simulink model "semi_solarwind"  (R2023b)
settings: Solver=VariableStepAuto  StartTime=0.0  StopTime=5  RelTol=1e-3
undefined symbols (not defined in the file): D1, Delta, Ion, Lithium
libraries: spsSeriesRLCBranchLib x26, spsVoltageMeasurementLib x9, spsDiodeLib x8, dspsrcs4 x8, spsCurrentMeasurementLib x5, spsThreePhaseVIMeasurementLib x5, spsMosfetLib x4, spsPWMGeneratorDCDCLib x4, spsPVArrayLib x4, spsThreePhaseTransformerTwoWindingsLib x3, spsThreePhaseParallelRLCLoadLib x3, spsThreePhaseSeriesRLCBranchLib x3
(part 1 of 2)
settings Model: Creator=yeowy  LastModifiedBy=yeowy

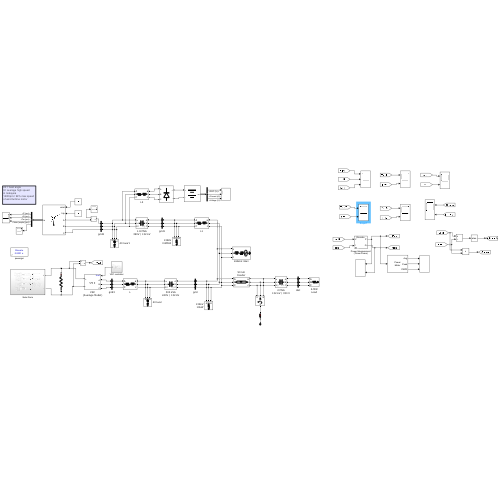
[thumbnail: Simulink's stored preview of the top-level diagram]
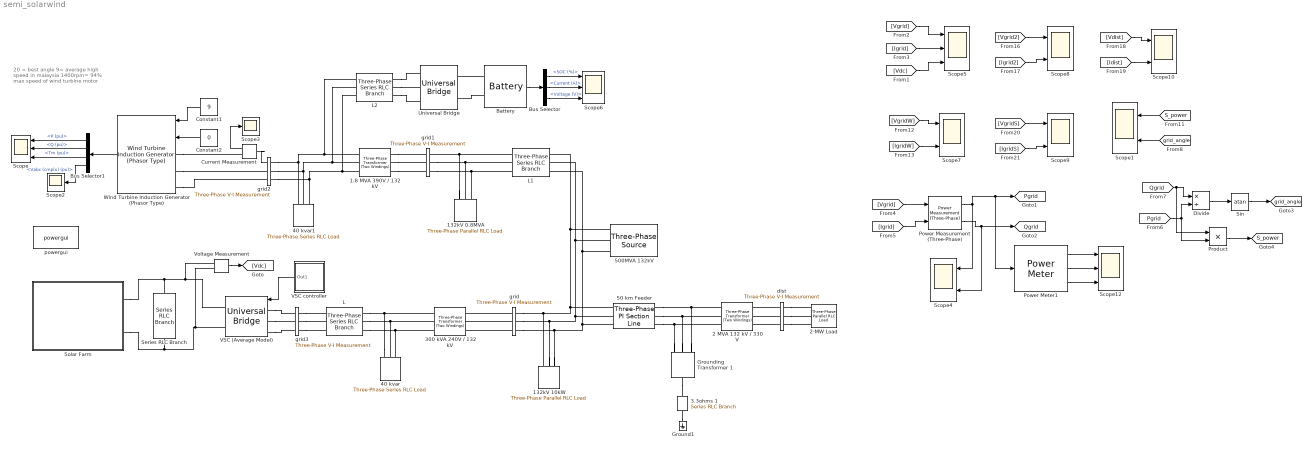
== system semi_solarwind ==
  note: 20 = best angle
      | 9= average high speed
      | in malaysia
      | 1400rpm= 94% max speed
      | of wind turbine motor
  1.8 MVA 390V / 132 kV : spsThreePhaseTransformerTwoWindingsLib/Three-Phase Transformer (Two Windings)  Winding1Connection=Yg  Winding2Connection=Delta (D1)  CoreType=Three single-phase transformers  SetSaturation=off  Hysteresis=off  DataFile='hysteresis'  SetInitialFlux=off  Measurements=None  UNITS=pu  NominalPower=[1.8e6 , 50 ]  Winding1=[ 132e3 , 0.001 , 0.03 ]  Winding2=[ 390 , 0.001 , 0.03 ]  Rm=500  Lm=500  L0=0.5  Saturation=[ 0,0 ; 0.0024,1.2 ; 1.0,1.52 ]  InitialFluxes=[ 0.8 , -0.8 , 0.7 ]  BreakLoop=off  DiscreteSolver=Trapezoidal iterative  DataType=off  TransfoNumber=0
  132kV 0.8MVA : spsThreePhaseParallelRLCLoadLib/Three-Phase Parallel RLC Load  LConnTagsString=A|B|C  Configuration=Y (grounded)  NominalVoltage=132e3  Vabc=[1e3 1e3 1e3]  Vabcp=[1e3 1e3 1e3]  NominalFrequency=50  UnbalancedPower=off  ActivePower=0.8e6  InductivePower=0  CapacitivePower=0  Pabc=[10e3 9e3 11e3]  QLabc=[100 90 110]  QCabc=[100 90 110]  Pabcp=[10e3 9e3 11e3]  QLabcp=[100 90 110]  QCabcp=[100 90 110]  Measurements=None  LoadType=constant Z
  132kV 10kW : spsThreePhaseParallelRLCLoadLib/Three-Phase Parallel RLC Load  LConnTagsString=A|B|C  Configuration=Y (grounded)  NominalVoltage=132e3  Vabc=[1e3 1e3 1e3]  Vabcp=[1e3 1e3 1e3]  NominalFrequency=50  UnbalancedPower=off  ActivePower=10e3  InductivePower=0  CapacitivePower=0  Pabc=[10e3 9e3 11e3]  QLabc=[100 90 110]  QCabc=[100 90 110]  Pabcp=[10e3 9e3 11e3]  QLabcp=[100 90 110]  QCabcp=[100 90 110]  Measurements=None  LoadType=constant Z
  2 MVA 132 kV / 330 V : spsThreePhaseTransformerTwoWindingsLib/Three-Phase Transformer (Two Windings)  Winding1Connection=Delta (D1)  Winding2Connection=Yg  CoreType=Three single-phase transformers  SetSaturation=off  Hysteresis=off  DataFile='hysteresis'  SetInitialFlux=off  Measurements=None  UNITS=pu  NominalPower=[2e6 , 50 ]  Winding1=[ 330 , 0.001 , 0.03 ]  Winding2=[ 132e3 , 0.001 , 0.03 ]  Rm=500  Lm=500  L0=0.5  Saturation=[ 0,0 ; 0.0024,1.2 ; 1.0,1.52 ]  InitialFluxes=[0.79999 -0.79999 0.70002]  BreakLoop=off  DiscreteSolver=Trapezoidal iterative  DataType=off  TransfoNumber=0
  2-MW Load : spsThreePhaseParallelRLCLoadLib/Three-Phase Parallel RLC Load  LConnTagsString=A|B|C  Configuration=Y (grounded)  NominalVoltage=240  Vabc=[1e3 1e3 1e3]  Vabcp=[1e3 1e3 1e3]  NominalFrequency=50  UnbalancedPower=off  ActivePower=2e6  InductivePower=0  CapacitivePower=0  Pabc=[10e3 9e3 11e3]  QLabc=[100 90 110]  QCabc=[100 90 110]  Pabcp=[10e3 9e3 11e3]  QLabcp=[100 90 110]  QCabcp=[100 90 110]  Measurements=None  LoadType=constant Z
  3.3ohms 1 : spsSeriesRLCBranchLib/Series RLC Branch  LConnTagsString=__new0  RConnTagsString=__new0  BranchType=R  Resistance=3.3  Inductance=[]  SetiL0=off  InitialCurrent=0  Capacitance=[]  Setx0=off  InitialVoltage=0  Measurements=None
  300 kVA 240V / 132 kV : spsThreePhaseTransformerTwoWindingsLib/Three-Phase Transformer (Two Windings)  Winding1Connection=Yg  Winding2Connection=Delta (D1)  CoreType=Three single-phase transformers  SetSaturation=off  Hysteresis=off  DataFile='hysteresis'  SetInitialFlux=off  Measurements=None  UNITS=pu  NominalPower=[0.3e6 , 50 ]  Winding1=[ 132e3 , 0.001 , 0.03 ]  Winding2=[ 240 , 0.001 , 0.03 ]  Rm=500  Lm=500  L0=0.5  Saturation=[ 0,0 ; 0.0024,1.2 ; 1.0,1.52 ]  InitialFluxes=[ 0.8 , -0.8 , 0.7 ]  BreakLoop=off  DiscreteSolver=Trapezoidal iterative  DataType=off  TransfoNumber=0
  40 kvar : spsThreePhaseSeriesRLCLoadLib/Three-Phase Series RLC Load  LConnTagsString=A|B|C  Configuration=Y (grounded)  NominalVoltage=240  Vabc=[1e3 1e3 1e3]  Vabcp=[1e3 1e3 1e3]  NominalFrequency=50  UnbalancedPower=off  ActivePower=400  InductivePower=0  CapacitivePower=400  Pabc=[10e3 9e3 11e3]  QLabc=[100 90 110]  QCabc=[100 90 110]  Pabcp=[10e3 9e3 11e3]  QLabcp=[100 90 110]  QCabcp=[100 90 110]  Measurements=None  LoadType=constant Z
  40 kvar1 : spsThreePhaseSeriesRLCLoadLib/Three-Phase Series RLC Load  LConnTagsString=A|B|C  Configuration=Y (grounded)  NominalVoltage=240  Vabc=[1e3 1e3 1e3]  Vabcp=[1e3 1e3 1e3]  NominalFrequency=50  UnbalancedPower=off  ActivePower=400  InductivePower=0  CapacitivePower=40e3  Pabc=[10e3 9e3 11e3]  QLabc=[100 90 110]  QCabc=[100 90 110]  Pabcp=[10e3 9e3 11e3]  QLabcp=[100 90 110]  QCabcp=[100 90 110]  Measurements=None  LoadType=constant Z
  50 km Feeder : spsThreePhasePISectionLineLib/Three-Phase PI Section Line  LConnTagsString=a|b|c  RConnTagsString=A|B|C  Length=50  Frequency=50  Resistances=[0.1153 0.413]  Inductances=[1.05e-3 3.32e-3]  Capacitances=[11.33e-009 5.01e-009]
  500MVA 132kV : spsThreePhaseSourceLib/Three-Phase Source  InternalConnection=Yg  VoltagePhases=off  Voltage=132e3  PhaseAngle=0  Voltage_phases=[25e3 25e3 25e3]/sqrt(3)  PhaseAngles_phases=[0 -120 +120]  Frequency=50  NonIdealSource=on  SpecifyImpedance=on  Resistance=0.8929  Inductance=16.58e-3  ShortCircuitLevel=500e6  BaseVoltage=132e3  XRratio=7  BusType=swing  Pref=10e3  Qref=0  Prefabc=[10e3, 10e3, 10e3]  Qrefabc=[0, 0, 0]  Qmin=-inf  Qmax=inf
  Battery : spsBatteryLib/Battery  BatType=Lithium-Ion  ShowTempParam=off  ThermalPreset=no  ShowAgeParam=off  NomV=240  NomQ=1e3  SOC=50  Batt_Tr=1  PresetModel=off  MaxQ=1000  MinV=235  FullV=255  Dis_rate=100  R=0.0023  Normal_OP=904.3478  expZone="[248.4887      49.13043]"  current=[6.5 13 32.5]  Units=Time  Tci=20  NomT=20  T2=-30  MaxQ2=4.8  FullV2=7.1  Normal_OP2=5.655  expZone2="[6.58           1]"  Rca=0.6  ti=2000  Dp=0  Neq0=0  Tsim=1e6  Ta1=25  Qeol=5.4*0.9  Reol=0.013333*1.2  Char_age=[2.3478, 3]  Dis_age=[2.3478, 10]  N1=1500  N2=10500  N3=1000  N4=1400  Ta2=45  N5=950
  Bus Selector : BusSelector  OutputSignals=SOC (%),Current (A),Voltage (V)
  Bus Selector1 : BusSelector  OutputSignals=P (pu),Q (pu),Tm (pu),Vabc (cmplx) (pu)
  Constant1 : Constant  Value=9
  Constant2 : Constant  Value=0
  Current Measurement : spsCurrentMeasurementLib/Current Measurement  PhasorSimulation=off  OutputType=Complex  PSBequivalent=0
  Divide : Product  Inputs=*/  RndMeth=Zero  SaturateOnIntegerOverflow=on
  Ground1 : spsGroundLib/Ground  LConnTagsString=a
  Grounding Transformer 1 : spsGroundingTransformerLib/Grounding Transformer   UNITS=pu  NominalPower="[100e6   50]"  NominalVoltage=132e3  ZeroSequenceImpedance_pu=[0.025 0.75]  MagnetizationBranch_pu=[500 500]  ZeroSequenceImpedance_SI=[0.052083 589.05]  MagnetizationBranch_SI=[1041.7 3.927e+005]  Measurements=None
  L : spsThreePhaseSeriesRLCBranchLib/Three-Phase Series RLC Branch  LConnTagsString=A|B|C  RConnTagsString=A|B|C  BranchType=RL  Resistance=1  Inductance=1e-4  Capacitance=inf  Measurements=None
  L1 : spsThreePhaseSeriesRLCBranchLib/Three-Phase Series RLC Branch  LConnTagsString=A|B|C  RConnTagsString=A|B|C  BranchType=RL  Resistance=1  Inductance=1e-4  Capacitance=inf  Measurements=None
  L2 : spsThreePhaseSeriesRLCBranchLib/Three-Phase Series RLC Branch  LConnTagsString=A|B|C  RConnTagsString=A|B|C  BranchType=RL  Resistance=1  Inductance=1e-6  Capacitance=inf  Measurements=None
  Power Measurement (Three-Phase) : eePowerMeasurement/Power Measurement (Three-Phase)  LabelModeActiveChoice=Discrete  F=50  K=[0 1]  Seq=Positive  Ts=0.01
  Power Meter1 : dspstat3/Power Meter  Measurement=All  ReferenceLoad=1  OutputPowerUnits=Watts  WindowLength=256  OverlapLength=255  AllowArbitraryInputLength=off  ComputeCCDF=off  PowerRange=50  PowerResolution=0.1  CCDFOutput=Relative power (dB above average power)  ProbabilityVector=[ 10; 1; 0.1; 0.01; 0.001; 0.0001 ]  RelativePowerVector=[ 0; 3; 6; 9; 12 ]  ResetPort=off  SimulateUsing=Code generation
  Product : Product
  Scope{,5..6,12} (4 alike) : Scope  NumInputPorts=3
  Scope{1,4,7..10} (6 alike) : Scope  NumInputPorts=2
  Scope2 : Scope
  Scope3 : Scope
  Series RLC Branch : spsSeriesRLCBranchLib/Series RLC Branch  LConnTagsString=__new0  RConnTagsString=__new0  BranchType=R  Resistance=0.5  Inductance=1e-3  SetiL0=off  InitialCurrent=0  Capacitance=1e-6  Setx0=off  InitialVoltage=0  Measurements=None
  Sin : Trigonometry  Operator=atan
  Solar Farm : Subsystem
  Universal Bridge : spsUniversalBridgeLib/Universal Bridge  Arms=3  SnubberResistance=1e5  SnubberCapacitance=inf  Device=Diodes  Ron=1e-3  Lon=0  ForwardVoltages="[  0  0  ]"  ForwardVoltage=0  GTOparameters=[ 10e-6 , 20e-6 ]  IGBTparameters=[ 1e-6 , 2e-6 ]  Measurements=None  Measurements_2=None  converterType=Rectifier
  VSC (Average Model) : spsUniversalBridgeLib/Universal Bridge  Arms=3  SnubberResistance=1e5  SnubberCapacitance=inf  Device=Average-model based VSC  Ron=1e-3  Lon=0  ForwardVoltages="[  0  0  ]"  ForwardVoltage=200  GTOparameters=[ 10e-6 , 20e-6 ]  IGBTparameters=[ 1e-6 , 2e-6 ]  Measurements=None  Measurements_2=None  converterType=Rectifier
  VSC controller : Subsystem
  Voltage Measurement : spsVoltageMeasurementLib/Voltage Measurement  PhasorSimulation=off  OutputType=Complex  PSBequivalent=0
  Wind Turbine Induction Generator (Phasor Type) : spsWindTurbineInductionGeneratorPhasorTypeLib/Wind Turbine Induction Generator (Phasor Type)  ExternalTm=off  nom=[1.8e6/0.9, 690, 50]  sta=[ 0.004843, 0.1248]  rot=[ 0.004377, 0.1791]  Lm=6.77  mec=[5.04, 0.01, 3]  init="[ -0.01,0,   0,0,0,   0,0,0 ]"  pitch_angle=0  Pmec=1.8e6  wind_base=9  speed_nom=1  P_wind_base=1  K_pitch_gain=[5 25]  pitch_max=45  pitch_rate=2
      settings: LibrarySourceBlock=|
      | sps_lib/Electrical Machines/Wind Turbine
      | Induction Generator
      | (Phasor Type)
  dist : spsThreePhaseVIMeasurementLib/Three-Phase V-I Measurement  VoltageMeasurement=phase-to-ground  SetLabelV=on  LabelV=Vdist  Vpu=off  VpuLL=off  CurrentMeasurement=yes  SetLabelI=on  LabelI=Idist  Ipu=off  Pbase=100e6  Vbase=500e3  OutputType=Magnitude  PhasorSimulation=off  PSBequivalent=0
  grid : spsThreePhaseVIMeasurementLib/Three-Phase V-I Measurement  VoltageMeasurement=phase-to-ground  SetLabelV=on  LabelV=Vgrid  Vpu=off  VpuLL=off  CurrentMeasurement=yes  SetLabelI=on  LabelI=Igrid  Ipu=off  Pbase=100e6  Vbase=500e3  OutputType=Magnitude  PhasorSimulation=off  PSBequivalent=0
  grid1 : spsThreePhaseVIMeasurementLib/Three-Phase V-I Measurement  VoltageMeasurement=phase-to-ground  SetLabelV=on  LabelV=Vgrid2  Vpu=off  VpuLL=off  CurrentMeasurement=yes  SetLabelI=on  LabelI=Igrid2  Ipu=off  Pbase=100e6  Vbase=500e3  OutputType=Magnitude  PhasorSimulation=off  PSBequivalent=0
  grid2 : spsThreePhaseVIMeasurementLib/Three-Phase V-I Measurement  VoltageMeasurement=phase-to-ground  SetLabelV=on  LabelV=VgridW  Vpu=off  VpuLL=off  CurrentMeasurement=yes  SetLabelI=on  LabelI=IgridW  Ipu=off  Pbase=100e6  Vbase=500e3  OutputType=Magnitude  PhasorSimulation=off  PSBequivalent=0
  grid3 : spsThreePhaseVIMeasurementLib/Three-Phase V-I Measurement  VoltageMeasurement=phase-to-ground  SetLabelV=on  LabelV=VgridS  Vpu=off  VpuLL=off  CurrentMeasurement=yes  SetLabelI=on  LabelI=IgridS  Ipu=off  Pbase=100e6  Vbase=500e3  OutputType=Magnitude  PhasorSimulation=off  PSBequivalent=0
  powergui : sps_lib/powergui  Priority=1  SimulationMode=Discrete  SampleTime=1e-4  frequency=50  Iterations=50  frequencyindice=0  Pbase=100e6  ErrMax=1e-4  UnitsV=kV  UnitsW=MW  buscounter=0  FunctionMessages=off  echomessages=off  EnableUseOfTLC=off  CurrentSourceSwitches=off  DisableSnubberDevices=off  DisableRonSwitches=off  DisableVfSwitches=off  DisplayEquations=off  AutomaticDiscreteSolvers=off  SolverType=Tustin/Backward Euler (TBE)  Interpol=off  ExternalGateDelay=off  methode=off  Ts=100  x0status=blocks  SPID=on  SwTol=0  HookPort=off  NonlinearTolerance=1e-4  nMaxIteration=100  ContinueOnMaxIteration=off  RestoreLinks=warning  ResistiveCurrentMeasurement=off  Frange=[0:2:500]  Ylog=off  Xlog=on  ShowGrid=off  save=off  variable=ZData  structure=0  ZoomFFT=off  StartTime=0.0  cycles=1  DisplayStyle=1  fundamental=60  FreqAxis=off  MaxFrequency=1000  frequencyindicesteady=1  RmsSteady=1  display=off
  tag scope: Pgrid=global, Qgrid=global, S_power=global, grid_angle=global
  wires:
  Voltage Measurement/1 -> [Vdc]
  [Vgrid] -> Power Measurement (Three-Phase)/1
  [Igrid] -> Power Measurement (Three-Phase)/2
  Power Measurement (Three-Phase)/2 -> Scope4/2, [Qgrid]
  Power Measurement (Three-Phase)/1 -> Scope4/1, Power Meter1/1, [Pgrid]
  [Qgrid] -> Product/1, Divide/1
  [Pgrid] -> Product/2, Divide/2
  Divide/1 -> Sin/1
  Sin/1 -> [grid_angle]
  Product/1 -> [S_power]
  [S_power] -> Scope1/1
  [grid_angle] -> Scope1/2
  VSC controller/1(Out1) -> VSC (Average Model)/1
  Constant2/1 -> Wind Turbine Induction Generator (Phasor Type)/2
  Bus Selector1/4 -> Scope2/1  "<Vabc (cmplx) (pu)>"
  Bus Selector1/3 -> Scope/3  "<Tm (pu)>"
  Bus Selector1/2 -> Scope/2  "<Q (pu)>"
  Bus Selector1/1 -> Scope/1  "<P (pu)>"
  Constant1/1 -> Wind Turbine Induction Generator (Phasor Type)/1
  Wind Turbine Induction Generator (Phasor Type)/1 -> Bus Selector1/1
  Battery/1 -> Bus Selector/1
  Current Measurement/1 -> Scope3/1
  Bus Selector/1 -> Scope6/1  "<SOC (%)>"
  Bus Selector/2 -> Scope6/2  "<Current (A)>"
  Bus Selector/3 -> Scope6/3  "<Voltage (V)>"
  [Vgrid] -> Scope5/1
  [Igrid] -> Scope5/2
  [Vdc] -> Scope5/3
  [VgridW] -> Scope7/1
  [IgridW] -> Scope7/2
  [Vgrid2] -> Scope8/1
  [Igrid2] -> Scope8/2
  [VgridS] -> Scope9/1
  [IgridS] -> Scope9/2
  [Idist] -> Scope10/2
  [Vdist] -> Scope10/1
  Power Meter1/1 -> Scope12/1
  Power Meter1/2 -> Scope12/2
  Power Meter1/3 -> Scope12/3
  connections:
  500MVA 132kV/RConn1 -- grid/RConn1 -- 132kV 10kW/LConn1 -- 50 km Feeder/LConn1 -- L1/RConn1
  500MVA 132kV/RConn3 -- 132kV 10kW/LConn3 -- grid/RConn3 -- 50 km Feeder/LConn3 -- L1/RConn3
  500MVA 132kV/RConn2 -- 132kV 10kW/LConn2 -- grid/RConn2 -- 50 km Feeder/LConn2 -- L1/RConn2
  grid/LConn3 -- 300 kVA 240V / 132 kV/LConn3
  grid/LConn2 -- 300 kVA 240V / 132 kV/LConn2
  grid/LConn1 -- 300 kVA 240V / 132 kV/LConn1
  40 kvar/LConn1 -- L/RConn1 -- 300 kVA 240V / 132 kV/RConn1
  L/RConn2 -- 300 kVA 240V / 132 kV/RConn2 -- 40 kvar/LConn2
  L/RConn3 -- 40 kvar/LConn3 -- 300 kVA 240V / 132 kV/RConn3
  1.8 MVA 390V / 132 kV/LConn1 -- grid1/LConn1
  1.8 MVA 390V / 132 kV/LConn2 -- grid1/LConn2
  1.8 MVA 390V / 132 kV/LConn3 -- grid1/LConn3
  40 kvar1/LConn1 -- L2/LConn1 -- 1.8 MVA 390V / 132 kV/RConn1 -- grid2/RConn1
  40 kvar1/LConn3 -- grid2/RConn3 -- L2/LConn3 -- 1.8 MVA 390V / 132 kV/RConn3
  40 kvar1/LConn2 -- grid2/RConn2 -- L2/LConn2 -- 1.8 MVA 390V / 132 kV/RConn2
  Series RLC Branch/LConn1 -- Solar Farm/RConn1 -- Voltage Measurement/LConn1 -- VSC (Average Model)/RConn1
  Series RLC Branch/RConn1 -- Solar Farm/RConn2 -- Voltage Measurement/LConn2 -- VSC (Average Model)/RConn2
  50 km Feeder/RConn1 -- Grounding Transformer 1/LConn1 -- 2 MVA 132 kV / 330 V/RConn1
  50 km Feeder/RConn2 -- Grounding Transformer 1/LConn2 -- 2 MVA 132 kV / 330 V/RConn2
  dist/LConn1 -- 2 MVA 132 kV / 330 V/LConn1
  dist/LConn2 -- 2 MVA 132 kV / 330 V/LConn2
  dist/LConn3 -- 2 MVA 132 kV / 330 V/LConn3
  dist/RConn3 -- 2-MW Load/LConn3
  dist/RConn2 -- 2-MW Load/LConn2
  dist/RConn1 -- 2-MW Load/LConn1
  VSC (Average Model)/LConn1 -- grid3/LConn1
  VSC (Average Model)/LConn2 -- grid3/LConn2
  VSC (Average Model)/LConn3 -- grid3/LConn3
  grid3/RConn1 -- L/LConn1
  grid3/RConn2 -- L/LConn2
  grid3/RConn3 -- L/LConn3
  Grounding Transformer 1/RConn1 -- 3.3ohms 1/LConn1
  3.3ohms 1/RConn1 -- Ground1/LConn1
  132kV 0.8MVA/LConn1 -- L1/LConn1 -- grid1/RConn1
  grid1/RConn2 -- L1/LConn2 -- 132kV 0.8MVA/LConn2
  grid1/RConn3 -- L1/LConn3 -- 132kV 0.8MVA/LConn3
  Battery/LConn1 -- Universal Bridge/RConn1
  Battery/LConn2 -- Universal Bridge/RConn2
  L2/RConn1 -- Universal Bridge/LConn1
  L2/RConn2 -- Universal Bridge/LConn2
  L2/RConn3 -- Universal Bridge/LConn3
  Wind Turbine Induction Generator (Phasor Type)/LConn1 -- Current Measurement/RConn1
  Wind Turbine Induction Generator (Phasor Type)/LConn2 -- grid2/LConn2
  Wind Turbine Induction Generator (Phasor Type)/LConn3 -- grid2/LConn3
  Current Measurement/LConn1 -- grid2/LConn1
  Grounding Transformer 1/LConn3 -- 50 km Feeder/RConn3 -- 2 MVA 132 kV / 330 V/RConn3

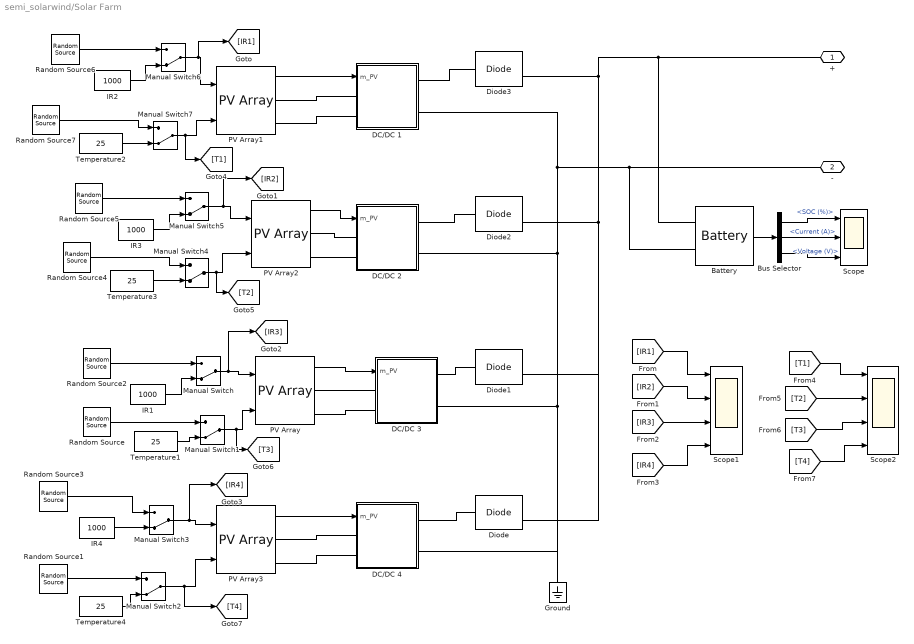
== system semi_solarwind/Solar Farm ==
  Battery : spsBatteryLib/Battery  BatType=Lithium-Ion  ShowTempParam=off  ThermalPreset=no  ShowAgeParam=off  NomV=680  NomQ=1e3  SOC=50  Batt_Tr=1  PresetModel=off  MaxQ=1000  MinV=660  FullV=690  Dis_rate=2000  R=0.0023  Normal_OP=904.3478  expZone="[688      49.13043]"  current=[6.5 13 32.5]  Units=Time  Tci=20  NomT=20  T2=-30  MaxQ2=4.8  FullV2=7.1  Normal_OP2=5.655  expZone2="[6.58           1]"  Rca=0.6  ti=2000  Dp=0  Neq0=0  Tsim=1e6  Ta1=25  Qeol=5.4*0.9  Reol=0.013333*1.2  Char_age=[2.3478, 3]  Dis_age=[2.3478, 10]  N1=1500  N2=10500  N3=1000  N4=1400  Ta2=45  N5=950
  Bus Selector : BusSelector  OutputSignals=SOC (%),Current (A),Voltage (V)
  DC/DC 1 : Subsystem
  DC/DC 2 : Subsystem
  DC/DC 3 : Subsystem
  DC/DC 4 : Subsystem
  Diode{,1..3} (4 alike) : spsDiodeLib/Diode  Ron=0.001  Lon=0  Vf=0.8  IC=0  UseSnubber=0  Rs=500  Cs=250e-9  Measurements=on
  Ground : spsGroundLib/Ground  LConnTagsString=a
  IR{1..4} (4 alike) : Constant  Value=1000
  Manual Switch{,1..7} (8 alike) : ManualSwitch  CurrentSetting=0
  PV Array{,1..3} (4 alike) : spsPVArrayLib/PV Array  Npar=65  Nser=20  PlotType=array @ 1000 W/m2 & specified temperatures  S_vec="[ 1000  500  100 ]"  Temp_C_vec="[ 60 45 25  ]"  ModuleName=Aavid Solar ASMS-270P  PlotWhenSelected=off  Pm=269.919  Ncell=72  Voc=44.5  Isc=8.42  Vm=35.1  Im=7.69  beta_Voc_pc=-0.3631  alpha_Isc_pc=0.084299  beta_Voc=-0.16158  alpha_Isc=0.007098  IL=8.4561  I0=3.263e-10  nI=1.0051  Rsh=121.6253  Rs=0.52087  RobustModel=off  RobustCellTemperature=313.3991  BAL=on  Tc=1e-6  Tfilter=5e-5
  Random Source{,1,4,7} (4 alike) : dspsrcs4/Random Source  SrcType=Uniform  NormMethod=Ziggurat  CltLength=12  MinVal=25  MaxVal=50  MeanVal=0  VarVal=1  RepMode=Not repeatable  rawSeed=1  IsInherit=off  SampMode=Discrete  SampTime=0.5  SampFrame=1  DataType=Double  OutComplex=Real  OutputFrames=off
  Random Source{2..3,5..6} (4 alike) : dspsrcs4/Random Source  SrcType=Uniform  NormMethod=Ziggurat  CltLength=12  MinVal=200  MaxVal=1000  MeanVal=0  VarVal=1  RepMode=Not repeatable  rawSeed=1  IsInherit=off  SampMode=Discrete  SampTime=0.5  SampFrame=1  DataType=Double  OutComplex=Real  OutputFrames=off
  Scope : Scope  NumInputPorts=3
  Scope1 : Scope  NumInputPorts=4
  Scope2 : Scope  NumInputPorts=4
  Temperature{1..4} (4 alike) : Constant  Value=25
  " +" : PMIOPort  Side=Right
  " -" : PMIOPort  Port=2  Side=Right
  wires:
  PV Array/1 -> DC/DC 3/1(m_PV)
  Manual Switch/1 -> [IR3], PV Array/1
  Random Source2/1 -> Manual Switch/1
  IR1/1 -> Manual Switch/2
  PV Array1/1 -> DC/DC 1/1(m_PV)
  PV Array2/1 -> DC/DC 2/1(m_PV)
  PV Array3/1 -> DC/DC 4/1(m_PV)
  Battery/1 -> Bus Selector/1
  Bus Selector/2 -> Scope/2  "<Current (A)>"
  Bus Selector/1 -> Scope/1  "<SOC (%)>"
  Bus Selector/3 -> Scope/3  "<Voltage (V)>"
  Temperature1/1 -> Manual Switch1/2
  Manual Switch1/1 -> [T3], PV Array/2
  Random Source/1 -> Manual Switch1/1
  Temperature4/1 -> Manual Switch2/2
  Random Source1/1 -> Manual Switch2/1
  Manual Switch2/1 -> [T4], PV Array3/2
  Random Source3/1 -> Manual Switch3/1
  IR4/1 -> Manual Switch3/2
  Manual Switch3/1 -> [IR4], PV Array3/1
  Temperature3/1 -> Manual Switch4/2
  Random Source4/1 -> Manual Switch4/1
  Manual Switch4/1 -> [T2], PV Array2/2
  Random Source5/1 -> Manual Switch5/1
  IR3/1 -> Manual Switch5/2
  Manual Switch5/1 -> [IR2], PV Array2/1
  Random Source6/1 -> Manual Switch6/1
  IR2/1 -> Manual Switch6/2
  Manual Switch6/1 -> [IR1], PV Array1/1
  Random Source7/1 -> Manual Switch7/1
  Temperature2/1 -> Manual Switch7/2
  Manual Switch7/1 -> [T1], PV Array1/2
  [IR4] -> Scope1/4
  [IR3] -> Scope1/3
  [IR2] -> Scope1/2
  [IR1] -> Scope1/1
  [T1] -> Scope2/1
  [T2] -> Scope2/2
  [T3] -> Scope2/3
  [T4] -> Scope2/4
  connections:
  DC/DC 3/LConn1 -- PV Array/RConn1
  DC/DC 3/LConn2 -- PV Array/RConn2
  PV Array1/RConn1 -- DC/DC 1/LConn1
  PV Array1/RConn2 -- DC/DC 1/LConn2
  DC/DC 4/LConn1 -- PV Array3/RConn1
  DC/DC 4/LConn2 -- PV Array3/RConn2
  DC/DC 4/RConn1 -- Diode/LConn1
  DC/DC 1/RConn1 -- Diode3/LConn1
  DC/DC 3/RConn1 -- Diode1/LConn1
  DC/DC 2/RConn1 -- Diode2/LConn1
  Diode3/RConn1 -- Diode1/RConn1 -- Diode/RConn1 -- Diode2/RConn1 -- " +"/RConn1 -- Battery/LConn1
  DC/DC 2/LConn2 -- PV Array2/RConn2
  DC/DC 2/LConn1 -- PV Array2/RConn1
  DC/DC 1/RConn2 -- Ground/LConn1 -- DC/DC 4/RConn2 -- DC/DC 3/RConn2 -- DC/DC 2/RConn2 -- " -"/RConn1 -- Battery/LConn2

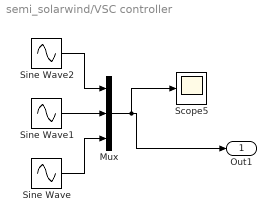
== system semi_solarwind/VSC controller ==
  Mux : Mux  Inputs=3
      settings: DisplayOption=signals
  Scope5 : Scope
  Sine Wave : Sin  Frequency=3.14*50  SampleTime=0
  Sine Wave1 : Sin  Frequency=3.14*50  Phase=4.1888  SampleTime=0
  Sine Wave2 : Sin  Frequency=3.14*50  Phase=2.0944  SampleTime=0
  Out1 : Outport
  wires:
  Sine Wave/1 -> Mux/3
  Mux/1 -> Scope5/1, Out1/1
  Sine Wave2/1 -> Mux/1
  Sine Wave1/1 -> Mux/2

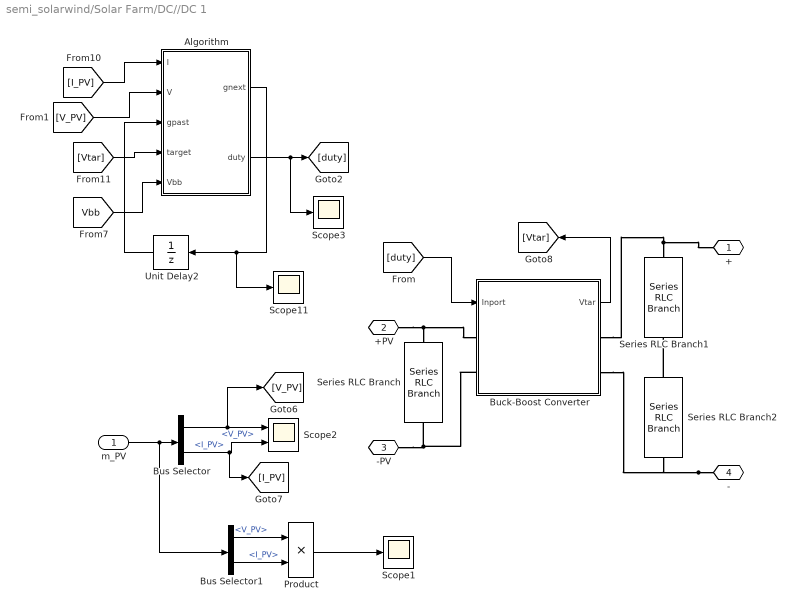
== system semi_solarwind/Solar Farm/DC//DC 1 ==
  m_PV : Inport
  Algorithm : MATLAB Function  TreatAsAtomicUnit=on
  Buck-Boost Converter : Subsystem
  Bus Selector : BusSelector  OutputSignals=V_PV,I_PV
  Bus Selector1 : BusSelector  OutputSignals=V_PV,I_PV
  Product : Product  RndMeth=Zero
  Scope1 : Scope
  Scope11 : Scope
  Scope2 : Scope  NumInputPorts=2
  Scope3 : Scope
  Series RLC Branch : spsSeriesRLCBranchLib/Series RLC Branch  LConnTagsString=__new0  RConnTagsString=__new0  BranchType=C  Resistance=1  Inductance=1e-3  SetiL0=off  InitialCurrent=0  Capacitance=1e-2  Setx0=off  InitialVoltage=0  Measurements=None
  Series RLC Branch1 : spsSeriesRLCBranchLib/Series RLC Branch  LConnTagsString=__new0  RConnTagsString=__new0  BranchType=C  Resistance=1  Inductance=1e-3  SetiL0=off  InitialCurrent=0  Capacitance=1e-6  Setx0=off  InitialVoltage=0  Measurements=None
  Series RLC Branch2 : spsSeriesRLCBranchLib/Series RLC Branch  LConnTagsString=__new0  RConnTagsString=__new0  BranchType=C  Resistance=1  Inductance=1e-3  SetiL0=off  InitialCurrent=0  Capacitance=1e-6  Setx0=off  InitialVoltage=0  Measurements=None
  Unit Delay2 : UnitDelay  InitialCondition=0.1  SampleTime=0.001  HasFrameUpgradeWarning=on
  " +" : PMIOPort  Side=Right
  +PV : PMIOPort  Port=2  Side=Left
  -PV : PMIOPort  Port=3  Side=Left
  " -" : PMIOPort  Port=4  Side=Right
  wires:
  Buck-Boost Converter/1(Vtar) -> [Vtar]
  [duty] -> Buck-Boost Converter/1(Inport)
  [Vbb] -> Algorithm/5(Vbb)
  Algorithm/1(gnext) -> Unit Delay2/1, Scope11/1
  [Vtar] -> Algorithm/4(target)
  [I_PV] -> Algorithm/1(I)
  Unit Delay2/1 -> Algorithm/3(gpast)
  Algorithm/2(duty) -> Scope3/1, [duty]
  [V_PV] -> Algorithm/2(V)
  Bus Selector1/2 -> Product/2  "<I_PV>"
  Bus Selector1/1 -> Product/1  "<V_PV>"
  Bus Selector/2 -> Scope2/2, [I_PV]  "<I_PV>"
  Bus Selector/1 -> Scope2/1, [V_PV]  "<V_PV>"
  m_PV/1 -> Bus Selector/1, Bus Selector1/1
  Product/1 -> Scope1/1
  connections:
  Series RLC Branch1/LConn1 -- " +"/RConn1 -- Buck-Boost Converter/RConn1
  Series RLC Branch2/LConn1 -- Series RLC Branch1/RConn1
  Series RLC Branch/LConn1 -- Buck-Boost Converter/LConn1 -- +PV/RConn1
  -PV/RConn1 -- Series RLC Branch/RConn1 -- Buck-Boost Converter/LConn2
  " -"/RConn1 -- Series RLC Branch2/RConn1 -- Buck-Boost Converter/RConn2

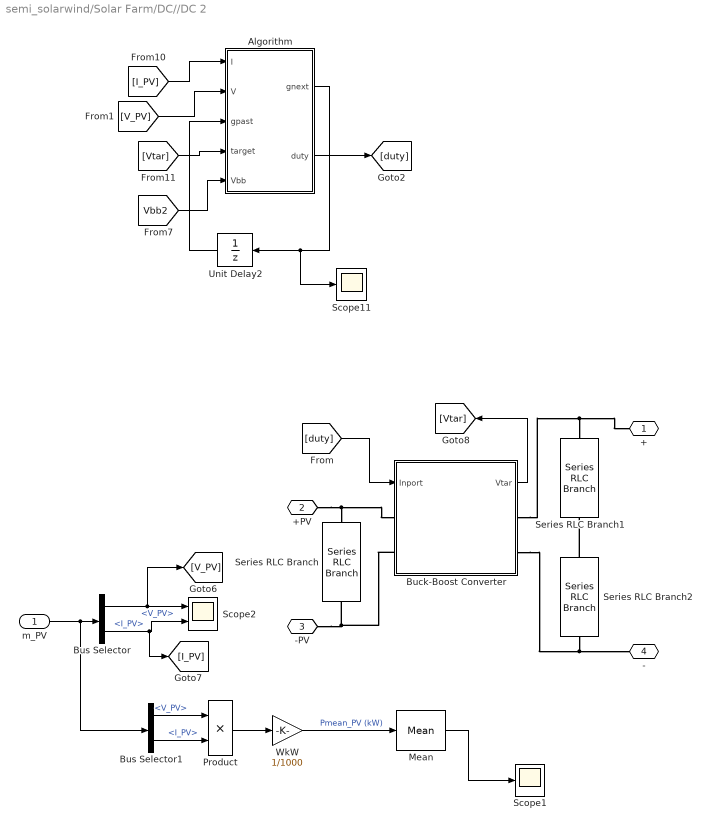
== system semi_solarwind/Solar Farm/DC//DC 2 ==
  m_PV : Inport
  Algorithm : MATLAB Function  TreatAsAtomicUnit=on
  Buck-Boost Converter : Subsystem
  Bus Selector : BusSelector  OutputSignals=V_PV,I_PV
  Bus Selector1 : BusSelector  OutputSignals=V_PV,I_PV
  Mean : spsMeanLib/Mean  Freq=60  Vinit=100  Ts=1e-4
  Product : Product  RndMeth=Zero
  Scope1 : Scope
  Scope11 : Scope
  Scope2 : Scope  NumInputPorts=2
  Series RLC Branch : spsSeriesRLCBranchLib/Series RLC Branch  LConnTagsString=__new0  RConnTagsString=__new0  BranchType=C  Resistance=1  Inductance=1e-3  SetiL0=off  InitialCurrent=0  Capacitance=1e-2  Setx0=off  InitialVoltage=0  Measurements=None
  Series RLC Branch1 : spsSeriesRLCBranchLib/Series RLC Branch  LConnTagsString=__new0  RConnTagsString=__new0  BranchType=C  Resistance=1  Inductance=1e-3  SetiL0=off  InitialCurrent=0  Capacitance=1e-6  Setx0=off  InitialVoltage=0  Measurements=None
  Series RLC Branch2 : spsSeriesRLCBranchLib/Series RLC Branch  LConnTagsString=__new0  RConnTagsString=__new0  BranchType=C  Resistance=1  Inductance=1e-3  SetiL0=off  InitialCurrent=0  Capacitance=1e-6  Setx0=off  InitialVoltage=0  Measurements=None
  Unit Delay2 : UnitDelay  InitialCondition=0.1  SampleTime=0.001  HasFrameUpgradeWarning=on
  WkW : Gain  Gain=1/1000
  " +" : PMIOPort  Side=Right
  +PV : PMIOPort  Port=2  Side=Left
  -PV : PMIOPort  Port=3  Side=Left
  " -" : PMIOPort  Port=4  Side=Right
  wires:
  m_PV/1 -> Bus Selector1/1, Bus Selector/1
  Bus Selector/1 -> [V_PV], Scope2/1  "<V_PV>"
  Bus Selector/2 -> [I_PV], Scope2/2  "<I_PV>"
  Bus Selector1/1 -> Product/1  "<V_PV>"
  Product/1 -> WkW/1
  Bus Selector1/2 -> Product/2  "<I_PV>"
  WkW/1 -> Mean/1  "Pmean_PV (kW)"
  Mean/1 -> Scope1/1
  [V_PV] -> Algorithm/2(V)
  Algorithm/2(duty) -> [duty]
  Unit Delay2/1 -> Algorithm/3(gpast)
  [I_PV] -> Algorithm/1(I)
  [Vtar] -> Algorithm/4(target)
  Algorithm/1(gnext) -> Scope11/1, Unit Delay2/1
  [Vbb2] -> Algorithm/5(Vbb)
  [duty] -> Buck-Boost Converter/1(Inport)
  Buck-Boost Converter/1(Vtar) -> [Vtar]
  connections:
  Buck-Boost Converter/RConn2 -- Series RLC Branch2/RConn1 -- " -"/RConn1
  Buck-Boost Converter/LConn2 -- Series RLC Branch/RConn1 -- -PV/RConn1
  +PV/RConn1 -- Buck-Boost Converter/LConn1 -- Series RLC Branch/LConn1
  Series RLC Branch2/LConn1 -- Series RLC Branch1/RConn1
  Buck-Boost Converter/RConn1 -- " +"/RConn1 -- Series RLC Branch1/LConn1

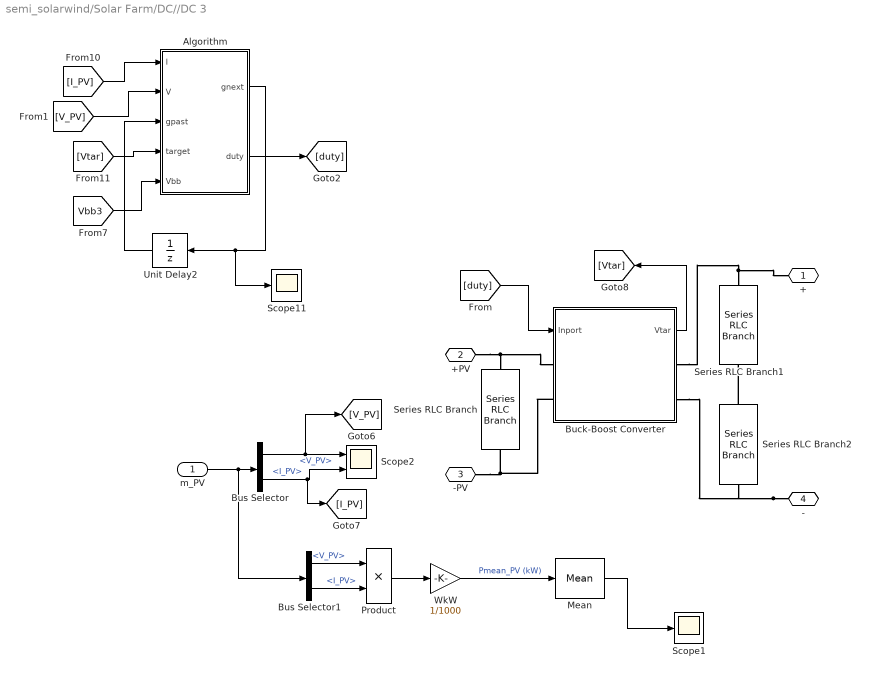
== system semi_solarwind/Solar Farm/DC//DC 3 ==
  m_PV : Inport
  Algorithm : MATLAB Function  TreatAsAtomicUnit=on
  Buck-Boost Converter : Subsystem
  Bus Selector : BusSelector  OutputSignals=V_PV,I_PV
  Bus Selector1 : BusSelector  OutputSignals=V_PV,I_PV
  Mean : spsMeanLib/Mean  Freq=60  Vinit=100  Ts=1e-4
  Product : Product  RndMeth=Zero
  Scope1 : Scope
  Scope11 : Scope
  Scope2 : Scope  NumInputPorts=2
  Series RLC Branch : spsSeriesRLCBranchLib/Series RLC Branch  LConnTagsString=__new0  RConnTagsString=__new0  BranchType=C  Resistance=1  Inductance=1e-3  SetiL0=off  InitialCurrent=0  Capacitance=1e-2  Setx0=off  InitialVoltage=0  Measurements=None
  Series RLC Branch1 : spsSeriesRLCBranchLib/Series RLC Branch  LConnTagsString=__new0  RConnTagsString=__new0  BranchType=C  Resistance=1  Inductance=1e-3  SetiL0=off  InitialCurrent=0  Capacitance=1e-6  Setx0=off  InitialVoltage=0  Measurements=None
  Series RLC Branch2 : spsSeriesRLCBranchLib/Series RLC Branch  LConnTagsString=__new0  RConnTagsString=__new0  BranchType=C  Resistance=1  Inductance=1e-3  SetiL0=off  InitialCurrent=0  Capacitance=1e-6  Setx0=off  InitialVoltage=0  Measurements=None
  Unit Delay2 : UnitDelay  InitialCondition=0.1  SampleTime=0.001  HasFrameUpgradeWarning=on
  WkW : Gain  Gain=1/1000
  " +" : PMIOPort  Side=Right
  +PV : PMIOPort  Port=2  Side=Left
  -PV : PMIOPort  Port=3  Side=Left
  " -" : PMIOPort  Port=4  Side=Right
  wires:
  Buck-Boost Converter/1(Vtar) -> [Vtar]
  [duty] -> Buck-Boost Converter/1(Inport)
  [Vbb3] -> Algorithm/5(Vbb)
  Algorithm/1(gnext) -> Unit Delay2/1, Scope11/1
  [Vtar] -> Algorithm/4(target)
  [I_PV] -> Algorithm/1(I)
  Unit Delay2/1 -> Algorithm/3(gpast)
  Algorithm/2(duty) -> [duty]
  [V_PV] -> Algorithm/2(V)
  Mean/1 -> Scope1/1
  WkW/1 -> Mean/1  "Pmean_PV (kW)"
  Bus Selector1/2 -> Product/2  "<I_PV>"
  Product/1 -> WkW/1
  Bus Selector1/1 -> Product/1  "<V_PV>"
  Bus Selector/2 -> Scope2/2, [I_PV]  "<I_PV>"
  Bus Selector/1 -> Scope2/1, [V_PV]  "<V_PV>"
  m_PV/1 -> Bus Selector/1, Bus Selector1/1
  connections:
  Series RLC Branch1/LConn1 -- " +"/RConn1 -- Buck-Boost Converter/RConn1
  Series RLC Branch2/LConn1 -- Series RLC Branch1/RConn1
  Series RLC Branch/LConn1 -- Buck-Boost Converter/LConn1 -- +PV/RConn1
  -PV/RConn1 -- Series RLC Branch/RConn1 -- Buck-Boost Converter/LConn2
  " -"/RConn1 -- Series RLC Branch2/RConn1 -- Buck-Boost Converter/RConn2

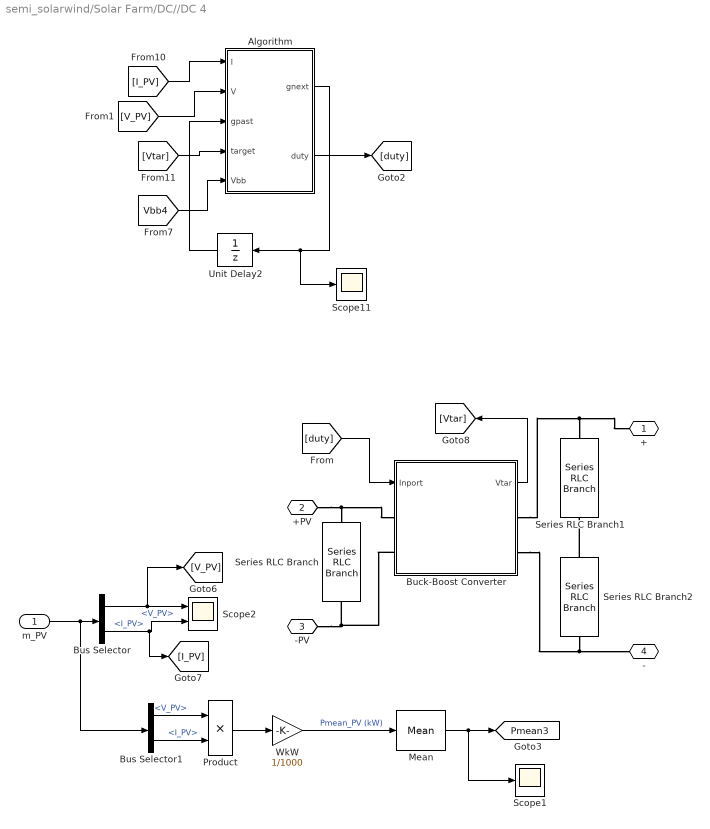
== system semi_solarwind/Solar Farm/DC//DC 4 ==
  m_PV : Inport
  Algorithm : MATLAB Function  TreatAsAtomicUnit=on
  Buck-Boost Converter : Subsystem
  Bus Selector : BusSelector  OutputSignals=V_PV,I_PV
  Bus Selector1 : BusSelector  OutputSignals=V_PV,I_PV
  Mean : spsMeanLib/Mean  Freq=60  Vinit=100  Ts=1e-4
  Product : Product  RndMeth=Zero
  Scope1 : Scope
  Scope11 : Scope
  Scope2 : Scope  NumInputPorts=2
  Series RLC Branch : spsSeriesRLCBranchLib/Series RLC Branch  LConnTagsString=__new0  RConnTagsString=__new0  BranchType=C  Resistance=1  Inductance=1e-3  SetiL0=off  InitialCurrent=0  Capacitance=1e-2  Setx0=off  InitialVoltage=0  Measurements=None
  Series RLC Branch1 : spsSeriesRLCBranchLib/Series RLC Branch  LConnTagsString=__new0  RConnTagsString=__new0  BranchType=C  Resistance=1  Inductance=1e-3  SetiL0=off  InitialCurrent=0  Capacitance=1e-6  Setx0=off  InitialVoltage=0  Measurements=None
  Series RLC Branch2 : spsSeriesRLCBranchLib/Series RLC Branch  LConnTagsString=__new0  RConnTagsString=__new0  BranchType=C  Resistance=1  Inductance=1e-3  SetiL0=off  InitialCurrent=0  Capacitance=1e-6  Setx0=off  InitialVoltage=0  Measurements=None
  Unit Delay2 : UnitDelay  InitialCondition=0.1  SampleTime=0.001  HasFrameUpgradeWarning=on
  WkW : Gain  Gain=1/1000
  " +" : PMIOPort  Side=Right
  +PV : PMIOPort  Port=2  Side=Left
  -PV : PMIOPort  Port=3  Side=Left
  " -" : PMIOPort  Port=4  Side=Right
  tag scope: Pmean3=global
  wires:
  m_PV/1 -> Bus Selector1/1, Bus Selector/1
  Bus Selector/1 -> [V_PV], Scope2/1  "<V_PV>"
  Bus Selector/2 -> [I_PV], Scope2/2  "<I_PV>"
  Bus Selector1/1 -> Product/1  "<V_PV>"
  Product/1 -> WkW/1
  Bus Selector1/2 -> Product/2  "<I_PV>"
  WkW/1 -> Mean/1  "Pmean_PV (kW)"
  Mean/1 -> Scope1/1, [Pmean3]
  [V_PV] -> Algorithm/2(V)
  Algorithm/2(duty) -> [duty]
  Unit Delay2/1 -> Algorithm/3(gpast)
  [I_PV] -> Algorithm/1(I)
  [Vtar] -> Algorithm/4(target)
  Algorithm/1(gnext) -> Scope11/1, Unit Delay2/1
  [Vbb4] -> Algorithm/5(Vbb)
  [duty] -> Buck-Boost Converter/1(Inport)
  Buck-Boost Converter/1(Vtar) -> [Vtar]
  connections:
  Buck-Boost Converter/RConn2 -- Series RLC Branch2/RConn1 -- " -"/RConn1
  Buck-Boost Converter/LConn2 -- Series RLC Branch/RConn1 -- -PV/RConn1
  +PV/RConn1 -- Buck-Boost Converter/LConn1 -- Series RLC Branch/LConn1
  Series RLC Branch2/LConn1 -- Series RLC Branch1/RConn1
  Buck-Boost Converter/RConn1 -- " +"/RConn1 -- Series RLC Branch1/LConn1

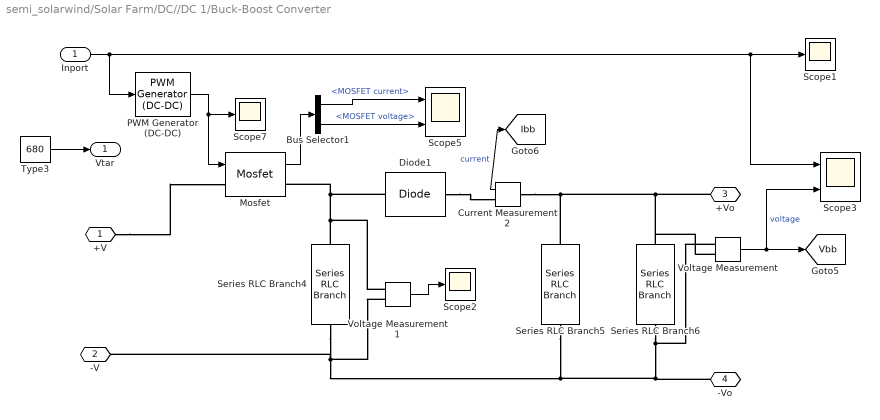
== system semi_solarwind/Solar Farm/DC//DC 1/Buck-Boost Converter ==
  Inport : Inport
  Bus Selector1 : BusSelector  OutputSignals=MOSFET current,MOSFET voltage
  Current Measurement2 : spsCurrentMeasurementLib/Current Measurement  PhasorSimulation=off  OutputType=Complex  PSBequivalent=0
  Diode1 : spsDiodeLib/Diode  Ron=0.001  Lon=0  Vf=0.8  IC=0  UseSnubber=0  Rs=500  Cs=250e-9  Measurements=off
  Mosfet : spsMosfetLib/Mosfet  Ron=0.1  Lon=0  Rd=0.01  Vfd=0  IC=0  Rs=1e5  Cs=inf  Measurements=on
  PWM Generator (DC-DC) : spsPWMGeneratorDCDCLib/PWM Generator (DC-DC)  Fsw=900  Ts=0
  Scope1 : Scope
  Scope2 : Scope
  Scope3 : Scope  NumInputPorts=2
  Scope5 : Scope  NumInputPorts=2
  Scope7 : Scope
  Series RLC Branch4 : spsSeriesRLCBranchLib/Series RLC Branch  LConnTagsString=__new0  RConnTagsString=__new0  BranchType=L  Resistance=1  Inductance=1e-3  SetiL0=off  InitialCurrent=0  Capacitance=1e-6  Setx0=off  InitialVoltage=0  Measurements=None
  Series RLC Branch5 : spsSeriesRLCBranchLib/Series RLC Branch  LConnTagsString=__new0  RConnTagsString=__new0  BranchType=C  Resistance=1  Inductance=1e-3  SetiL0=off  InitialCurrent=0  Capacitance=1e-2  Setx0=off  InitialVoltage=0  Measurements=None
  Series RLC Branch6 : spsSeriesRLCBranchLib/Series RLC Branch  LConnTagsString=__new0  RConnTagsString=__new0  BranchType=R  Resistance=50  Inductance=1e-3  SetiL0=off  InitialCurrent=0  Capacitance=1e-6  Setx0=off  InitialVoltage=0  Measurements=None
  Type3 : Constant  Value=680  SampleTime=0
  Voltage Measurement : spsVoltageMeasurementLib/Voltage Measurement  PhasorSimulation=off  OutputType=Complex  PSBequivalent=0
  Voltage Measurement1 : spsVoltageMeasurementLib/Voltage Measurement  PhasorSimulation=off  OutputType=Complex  PSBequivalent=0
  +V : PMIOPort  Side=Left
  -V : PMIOPort  Port=2  Side=Left
  +Vo : PMIOPort  Port=3  Side=Right
  -Vo : PMIOPort  Port=4  Side=Right
  Vtar : Outport
  tag scope: Ibb=global, Vbb=global
  wires:
  Inport/1 -> Scope3/1, Scope1/1, PWM Generator (DC-DC)/1
  Mosfet/1 -> Bus Selector1/1
  PWM Generator (DC-DC)/1 -> Scope7/1, Mosfet/1
  Type3/1 -> Vtar/1
  Current Measurement2/1 -> [Ibb]  "current"
  Bus Selector1/2 -> Scope5/2  "<MOSFET voltage>"
  Voltage Measurement1/1 -> Scope2/1
  Bus Selector1/1 -> Scope5/1  "<MOSFET current>"
  Voltage Measurement/1 -> Scope3/2, [Vbb]  "voltage"
  connections:
  +V/RConn1 -- Mosfet/LConn1
  Diode1/LConn1 -- Current Measurement2/RConn1
  Current Measurement2/LConn1 -- Series RLC Branch6/LConn1 -- Voltage Measurement/LConn2 -- +Vo/RConn1 -- Series RLC Branch5/RConn1
  Series RLC Branch4/LConn1 -- Voltage Measurement1/LConn1 -- Diode1/RConn1 -- Mosfet/RConn1
  Voltage Measurement/LConn1 -- Series RLC Branch5/LConn1 -- Voltage Measurement1/LConn2 -- -V/RConn1 -- Series RLC Branch4/RConn1 -- -Vo/RConn1 -- Series RLC Branch6/RConn1

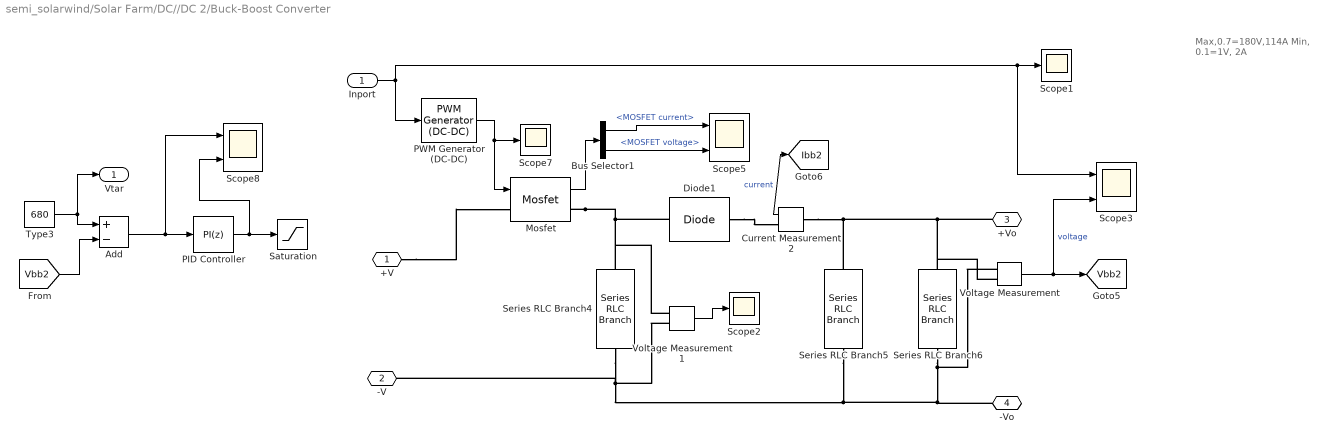
== system semi_solarwind/Solar Farm/DC//DC 2/Buck-Boost Converter ==
  note: Max,0.7=180V,114A
      | Min, 0.1=1V, 2A
  Inport : Inport
  Add : Sum  Inputs=+-
  Bus Selector1 : BusSelector  OutputSignals=MOSFET current,MOSFET voltage
  Current Measurement2 : spsCurrentMeasurementLib/Current Measurement  PhasorSimulation=off  OutputType=Complex  PSBequivalent=0
  Diode1 : spsDiodeLib/Diode  Ron=0.001  Lon=0  Vf=0.8  IC=0  UseSnubber=0  Rs=500  Cs=250e-9  Measurements=off
  Mosfet : spsMosfetLib/Mosfet  Ron=0.1  Lon=0  Rd=0.01  Vfd=0  IC=0  Rs=1e5  Cs=inf  Measurements=on
  PID Controller : slpidlib/PID Controller  Controller=PI  Form=Parallel  TimeDomain=Discrete-time  UseExternalTs=off  SampleTime=-1  IntegratorMethod=Forward Euler  FilterMethod=Forward Euler  ControllerParametersSource=internal  P=0.448206848938492  I=8.01083955194228  UseKiTs=off  D=0  N=100  UseFilter=on  TunerSelectOption=Transfer Function Based (PID Tuner App)  InitialConditionSource=internal  InitialConditionForIntegrator=0  InitialConditionForFilter=0  DifferentiatorICPrevScaledInput=0  ExternalReset=none  TrackingMode=off  Kt=1  LimitOutput=on  SatLimitsSource=internal  UpperSaturationLimit=0.8  LowerSaturationLimit=0  LinearizeAsGain=off  AntiWindupMode=none  Kb=1  LimitIntegrator=on  UpperIntegratorSaturationLimit=0.8  LowerIntegratorSaturationLimit=0  POutMin=[]  POutMax=[]  IOutMin=[]  IOutMax=[]  DOutMin=[]  DOutMax=[]  NOutMin=[]  NOutMax=[]  SumOutMin=[]  SumOutMax=[]  SaturationOutMin=[]  SaturationOutMax=[]  PParamMin=[]  PParamMax=[]  IParamMin=[]  IParamMax=[]  DParamMin=[]  DParamMax=[]  NParamMin=[]  NParamMax=[]  KbParamMin=[]  KbParamMax=[]  KtParamMin=[]  KtParamMax=[]  KbOutMin=[]  KbOutMax=[]  KtOutMin=[]  KtOutMax=[]  IntegratorOutMin=[]  IntegratorOutMax=[]  FilterOutMin=[]  FilterOutMax=[]  SumI1OutMin=[]  SumI1OutMax=[]  SumI2OutMin=[]  SumI2OutMax=[]  SumI3OutMin=[]  SumI3OutMax=[]  SumI4OutMin=[]  SumI4OutMax=[]  SumDOutMin=[]  SumDOutMax=[]  DifferentiatorOutMin=[]  DifferentiatorOutMax=[]  FilterDiffOutCoefMin=[]  FilterDiffOutCoefMax=[]  ReciprocalOutMin=[]  ReciprocalOutMax=[]  SumDenOutMin=[]  SumDenOutMax=[]  SumNumOutMin=[]  SumNumOutMax=[]  DivideOutMin=[]  DivideOutMax=[]  UdiffTsProdOutMin=[]  UdiffTsProdOutMax=[]  NTsProdOutMin=[]  NTsProdOutMax=[]  UintegralTsProdOutMin=[]  UintegralTsProdOutMax=[]  UngainTsProdOutMin=[]  UngainTsProdOutMax=[]  ClampingZeroOutDataTypeStr=Inherit: Inherit via back propagation  ClampingZeroOutMin=[]  ClampingZeroOutMax=[]  FilterDenConstantOutDataTypeStr=Inherit: Inherit via back propagation  FilterDenConstantOutMin=[]  FilterDenConstantOutMax=[]  PCopyOutDataTypeStr=Inherit: Inherit via back propagation  PCopyOutMin=[]  PCopyOutMax=[]  NCopyOutDataTypeStr=Inherit: Inherit via back propagation  NCopyOutMin=[]  NCopyOutMax=[]  IntegratorContinuousStateAttributes=''  IntegratorStateMustResolveToSignalObject=off  IntegratorRTWStateStorageClass=Auto  FilterContinuousStateAttributes=''  FilterStateMustResolveToSignalObject=off  FilterRTWStateStorageClass=Auto  ParallelPVariant=InternalParameters  IdealPVariant=Disabled  IVariant=InternalParameters  DVariant=Disabled  IntegratorVariant=Discrete  SatVariant=Enabled  AWVariant=Passthrough  PCopyVariant=Disabled  TRVariant=Disabled  FdbkBlocksVariant=Forward  IdealPFdbkVariant=Disabled  SatFdbkVariant=Disabled  DerivativeFilterVariant=Disabled  NVariant=Disabled  NCopyVariant=Disabled_SignalSpec  FilterICVariant=Disabled  IntegratorICVariant=InternalICs  ExternalResetVariant=Disabled  TRSumVariant=Passthrough  SumFdbkVariant=Disabled  SumVariant=Sum_PI  TsampFilterVariant=InternalTs  TsampNgainVariant=Passthrough  TsampIntegralVariant=Disabled_SignalSpec  ExternalSaturationOutDataTypeStr=Inherit: Same as second input
  PWM Generator (DC-DC) : spsPWMGeneratorDCDCLib/PWM Generator (DC-DC)  Fsw=900  Ts=0
  Saturation : Saturate  UpperLimit=0.8  LowerLimit=0
  Scope1 : Scope
  Scope2 : Scope
  Scope3 : Scope  NumInputPorts=2
  Scope5 : Scope  NumInputPorts=2
  Scope7 : Scope
  Scope8 : Scope  NumInputPorts=2
  Series RLC Branch4 : spsSeriesRLCBranchLib/Series RLC Branch  LConnTagsString=__new0  RConnTagsString=__new0  BranchType=L  Resistance=1  Inductance=1e-3  SetiL0=off  InitialCurrent=0  Capacitance=1e-6  Setx0=off  InitialVoltage=0  Measurements=None
  Series RLC Branch5 : spsSeriesRLCBranchLib/Series RLC Branch  LConnTagsString=__new0  RConnTagsString=__new0  BranchType=C  Resistance=1  Inductance=1e-3  SetiL0=off  InitialCurrent=0  Capacitance=1e-2  Setx0=off  InitialVoltage=0  Measurements=None
  Series RLC Branch6 : spsSeriesRLCBranchLib/Series RLC Branch  LConnTagsString=__new0  RConnTagsString=__new0  BranchType=R  Resistance=50  Inductance=1e-3  SetiL0=off  InitialCurrent=0  Capacitance=1e-6  Setx0=off  InitialVoltage=0  Measurements=None
  Type3 : Constant  Value=680  SampleTime=0
  Voltage Measurement : spsVoltageMeasurementLib/Voltage Measurement  PhasorSimulation=off  OutputType=Complex  PSBequivalent=0
  Voltage Measurement1 : spsVoltageMeasurementLib/Voltage Measurement  PhasorSimulation=off  OutputType=Complex  PSBequivalent=0
  +V : PMIOPort  Side=Left
  -V : PMIOPort  Port=2  Side=Left
  +Vo : PMIOPort  Port=3  Side=Right
  -Vo : PMIOPort  Port=4  Side=Right
  Vtar : Outport
  tag scope: Ibb2=global, Vbb2=global
  wires:
  [Vbb2] -> Add/2
  Voltage Measurement/1 -> Scope3/2, [Vbb2]  "voltage"
  Bus Selector1/1 -> Scope5/1  "<MOSFET current>"
  Voltage Measurement1/1 -> Scope2/1
  Bus Selector1/2 -> Scope5/2  "<MOSFET voltage>"
  PID Controller/1 -> Scope8/2, Saturation/1
  Add/1 -> Scope8/1, PID Controller/1
  Current Measurement2/1 -> [Ibb2]  "current"
  Type3/1 -> Vtar/1, Add/1
  PWM Generator (DC-DC)/1 -> Mosfet/1, Scope7/1
  Mosfet/1 -> Bus Selector1/1
  Inport/1 -> PWM Generator (DC-DC)/1, Scope3/1, Scope1/1
  connections:
  Series RLC Branch6/RConn1 -- -Vo/RConn1 -- Series RLC Branch4/RConn1 -- -V/RConn1 -- Voltage Measurement1/LConn2 -- Series RLC Branch5/LConn1 -- Voltage Measurement/LConn1
  Mosfet/RConn1 -- Diode1/RConn1 -- Voltage Measurement1/LConn1 -- Series RLC Branch4/LConn1
  Series RLC Branch5/RConn1 -- +Vo/RConn1 -- Voltage Measurement/LConn2 -- Series RLC Branch6/LConn1 -- Current Measurement2/LConn1
  Diode1/LConn1 -- Current Measurement2/RConn1
  +V/RConn1 -- Mosfet/LConn1

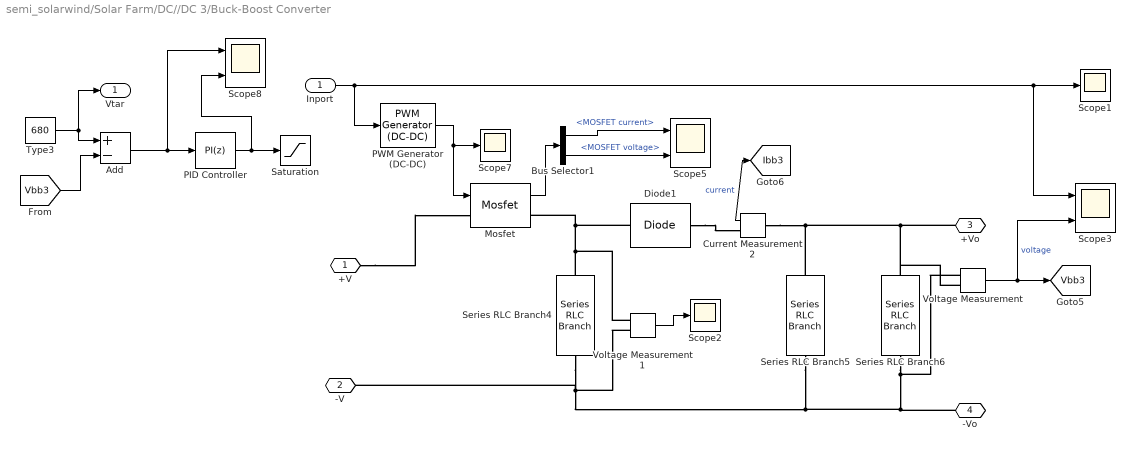
== system semi_solarwind/Solar Farm/DC//DC 3/Buck-Boost Converter ==
  Inport : Inport
  Add : Sum  Inputs=+-
  Bus Selector1 : BusSelector  OutputSignals=MOSFET current,MOSFET voltage
  Current Measurement2 : spsCurrentMeasurementLib/Current Measurement  PhasorSimulation=off  OutputType=Complex  PSBequivalent=0
  Diode1 : spsDiodeLib/Diode  Ron=0.001  Lon=0  Vf=0.8  IC=0  UseSnubber=0  Rs=500  Cs=250e-9  Measurements=off
  Mosfet : spsMosfetLib/Mosfet  Ron=0.1  Lon=0  Rd=0.01  Vfd=0  IC=0  Rs=1e5  Cs=inf  Measurements=on
  PID Controller : slpidlib/PID Controller  Controller=PI  Form=Parallel  TimeDomain=Discrete-time  UseExternalTs=off  SampleTime=-1  IntegratorMethod=Forward Euler  FilterMethod=Forward Euler  ControllerParametersSource=internal  P=0.448206848938492  I=8.01083955194228  UseKiTs=off  D=0  N=100  UseFilter=on  TunerSelectOption=Transfer Function Based (PID Tuner App)  InitialConditionSource=internal  InitialConditionForIntegrator=0  InitialConditionForFilter=0  DifferentiatorICPrevScaledInput=0  ExternalReset=none  TrackingMode=off  Kt=1  LimitOutput=on  SatLimitsSource=internal  UpperSaturationLimit=0.8  LowerSaturationLimit=0  LinearizeAsGain=off  AntiWindupMode=none  Kb=1  LimitIntegrator=on  UpperIntegratorSaturationLimit=0.8  LowerIntegratorSaturationLimit=0  POutMin=[]  POutMax=[]  IOutMin=[]  IOutMax=[]  DOutMin=[]  DOutMax=[]  NOutMin=[]  NOutMax=[]  SumOutMin=[]  SumOutMax=[]  SaturationOutMin=[]  SaturationOutMax=[]  PParamMin=[]  PParamMax=[]  IParamMin=[]  IParamMax=[]  DParamMin=[]  DParamMax=[]  NParamMin=[]  NParamMax=[]  KbParamMin=[]  KbParamMax=[]  KtParamMin=[]  KtParamMax=[]  KbOutMin=[]  KbOutMax=[]  KtOutMin=[]  KtOutMax=[]  IntegratorOutMin=[]  IntegratorOutMax=[]  FilterOutMin=[]  FilterOutMax=[]  SumI1OutMin=[]  SumI1OutMax=[]  SumI2OutMin=[]  SumI2OutMax=[]  SumI3OutMin=[]  SumI3OutMax=[]  SumI4OutMin=[]  SumI4OutMax=[]  SumDOutMin=[]  SumDOutMax=[]  DifferentiatorOutMin=[]  DifferentiatorOutMax=[]  FilterDiffOutCoefMin=[]  FilterDiffOutCoefMax=[]  ReciprocalOutMin=[]  ReciprocalOutMax=[]  SumDenOutMin=[]  SumDenOutMax=[]  SumNumOutMin=[]  SumNumOutMax=[]  DivideOutMin=[]  DivideOutMax=[]  UdiffTsProdOutMin=[]  UdiffTsProdOutMax=[]  NTsProdOutMin=[]  NTsProdOutMax=[]  UintegralTsProdOutMin=[]  UintegralTsProdOutMax=[]  UngainTsProdOutMin=[]  UngainTsProdOutMax=[]  ClampingZeroOutDataTypeStr=Inherit: Inherit via back propagation  ClampingZeroOutMin=[]  ClampingZeroOutMax=[]  FilterDenConstantOutDataTypeStr=Inherit: Inherit via back propagation  FilterDenConstantOutMin=[]  FilterDenConstantOutMax=[]  PCopyOutDataTypeStr=Inherit: Inherit via back propagation  PCopyOutMin=[]  PCopyOutMax=[]  NCopyOutDataTypeStr=Inherit: Inherit via back propagation  NCopyOutMin=[]  NCopyOutMax=[]  IntegratorContinuousStateAttributes=''  IntegratorStateMustResolveToSignalObject=off  IntegratorRTWStateStorageClass=Auto  FilterContinuousStateAttributes=''  FilterStateMustResolveToSignalObject=off  FilterRTWStateStorageClass=Auto  ParallelPVariant=InternalParameters  IdealPVariant=Disabled  IVariant=InternalParameters  DVariant=Disabled  IntegratorVariant=Discrete  SatVariant=Enabled  AWVariant=Passthrough  PCopyVariant=Disabled  TRVariant=Disabled  FdbkBlocksVariant=Forward  IdealPFdbkVariant=Disabled  SatFdbkVariant=Disabled  DerivativeFilterVariant=Disabled  NVariant=Disabled  NCopyVariant=Disabled_SignalSpec  FilterICVariant=Disabled  IntegratorICVariant=InternalICs  ExternalResetVariant=Disabled  TRSumVariant=Passthrough  SumFdbkVariant=Disabled  SumVariant=Sum_PI  TsampFilterVariant=InternalTs  TsampNgainVariant=Passthrough  TsampIntegralVariant=Disabled_SignalSpec  ExternalSaturationOutDataTypeStr=Inherit: Same as second input
  PWM Generator (DC-DC) : spsPWMGeneratorDCDCLib/PWM Generator (DC-DC)  Fsw=900  Ts=0
  Saturation : Saturate  UpperLimit=0.8  LowerLimit=0
  Scope1 : Scope
  Scope2 : Scope
  Scope3 : Scope  NumInputPorts=2
  Scope5 : Scope  NumInputPorts=2
  Scope7 : Scope
  Scope8 : Scope  NumInputPorts=2
  Series RLC Branch4 : spsSeriesRLCBranchLib/Series RLC Branch  LConnTagsString=__new0  RConnTagsString=__new0  BranchType=L  Resistance=1  Inductance=1e-3  SetiL0=off  InitialCurrent=0  Capacitance=1e-6  Setx0=off  InitialVoltage=0  Measurements=None
  Series RLC Branch5 : spsSeriesRLCBranchLib/Series RLC Branch  LConnTagsString=__new0  RConnTagsString=__new0  BranchType=C  Resistance=1  Inductance=1e-3  SetiL0=off  InitialCurrent=0  Capacitance=1e-2  Setx0=off  InitialVoltage=0  Measurements=None
  Series RLC Branch6 : spsSeriesRLCBranchLib/Series RLC Branch  LConnTagsString=__new0  RConnTagsString=__new0  BranchType=R  Resistance=50  Inductance=1e-3  SetiL0=off  InitialCurrent=0  Capacitance=1e-6  Setx0=off  InitialVoltage=0  Measurements=None
  Type3 : Constant  Value=680  SampleTime=0
  Voltage Measurement : spsVoltageMeasurementLib/Voltage Measurement  PhasorSimulation=off  OutputType=Complex  PSBequivalent=0
  Voltage Measurement1 : spsVoltageMeasurementLib/Voltage Measurement  PhasorSimulation=off  OutputType=Complex  PSBequivalent=0
  +V : PMIOPort  Side=Left
  -V : PMIOPort  Port=2  Side=Left
  +Vo : PMIOPort  Port=3  Side=Right
  -Vo : PMIOPort  Port=4  Side=Right
  Vtar : Outport
  tag scope: Ibb3=global, Vbb3=global
  wires:
  Inport/1 -> Scope3/1, Scope1/1, PWM Generator (DC-DC)/1
  Mosfet/1 -> Bus Selector1/1
  PWM Generator (DC-DC)/1 -> Scope7/1, Mosfet/1
  Type3/1 -> Add/1, Vtar/1
  Current Measurement2/1 -> [Ibb3]  "current"
  Add/1 -> PID Controller/1, Scope8/1
  PID Controller/1 -> Saturation/1, Scope8/2
  Bus Selector1/2 -> Scope5/2  "<MOSFET voltage>"
  Voltage Measurement1/1 -> Scope2/1
  Bus Selector1/1 -> Scope5/1  "<MOSFET current>"
  Voltage Measurement/1 -> Scope3/2, [Vbb3]  "voltage"
  [Vbb3] -> Add/2
  connections:
  +V/RConn1 -- Mosfet/LConn1
  Diode1/LConn1 -- Current Measurement2/RConn1
  Current Measurement2/LConn1 -- Series RLC Branch6/LConn1 -- Voltage Measurement/LConn2 -- +Vo/RConn1 -- Series RLC Branch5/RConn1
  Series RLC Branch4/LConn1 -- Voltage Measurement1/LConn1 -- Diode1/RConn1 -- Mosfet/RConn1
  Voltage Measurement/LConn1 -- Series RLC Branch5/LConn1 -- Voltage Measurement1/LConn2 -- -V/RConn1 -- Series RLC Branch4/RConn1 -- -Vo/RConn1 -- Series RLC Branch6/RConn1
